simulink model "height_control"  (R2022a)
settings: Solver=VariableStepAuto  StartTime=0.0  StopTime=10.0  RelTol=1e-3
settings Model: Creator=siddh  LastModifiedBy=siddh

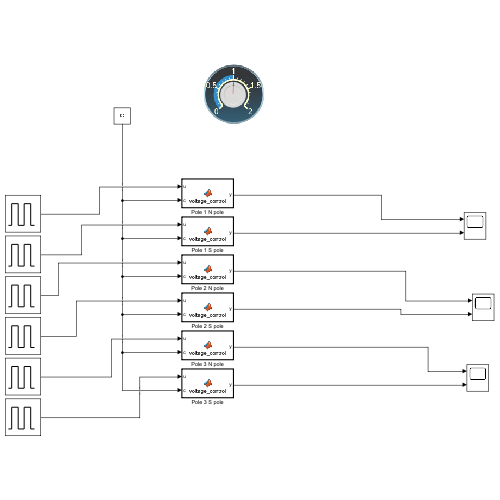
[thumbnail: Simulink's stored preview of the top-level diagram]
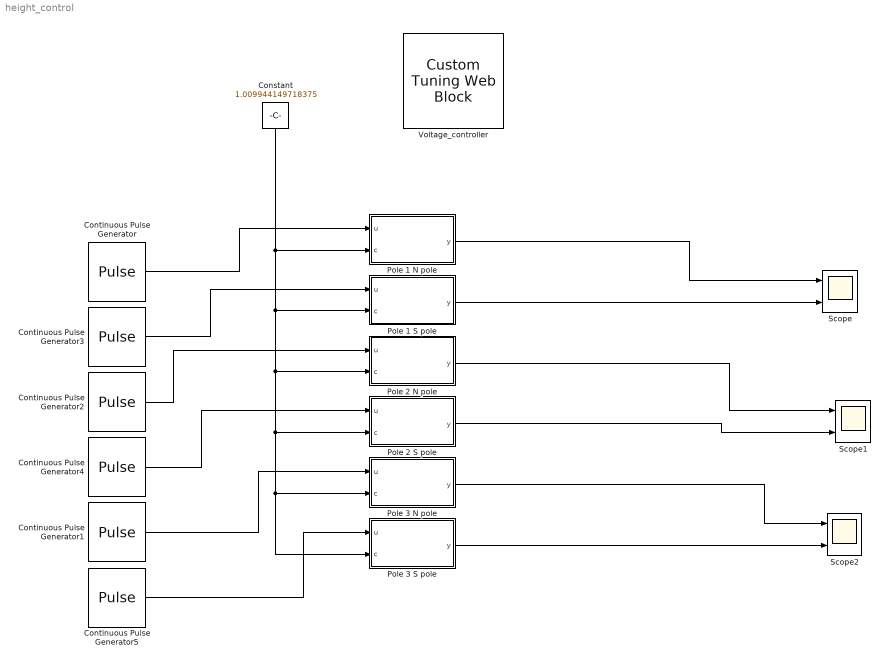
== system height_control ==
  Constant : Constant  Value=1.009944149718375
  Continuous Pulse Generator : DiscretePulseGenerator  PulseType=Time based  Period=3  PulseWidth=100/3
  Continuous Pulse Generator1 : DiscretePulseGenerator  PulseType=Time based  Period=3  PulseWidth=100/3  PhaseDelay=2
  Continuous Pulse Generator2 : DiscretePulseGenerator  PulseType=Time based  Period=3  PulseWidth=100/3  PhaseDelay=1
  Continuous Pulse Generator3 : DiscretePulseGenerator  PulseType=Time based  Amplitude=-1  Period=3  PulseWidth=100/3
  Continuous Pulse Generator4 : DiscretePulseGenerator  PulseType=Time based  Amplitude=-1  Period=3  PulseWidth=100/3  PhaseDelay=1
  Continuous Pulse Generator5 : DiscretePulseGenerator  PulseType=Time based  Amplitude=-1  Period=3  PulseWidth=100/3  PhaseDelay=2
  Pole 1 N pole : MATLAB Function  TreatAsAtomicUnit=on
  Pole 1 S pole : MATLAB Function  TreatAsAtomicUnit=on
  Pole 2 N pole : MATLAB Function  TreatAsAtomicUnit=on
  Pole 2 S pole : MATLAB Function  TreatAsAtomicUnit=on
  Pole 3 N pole : MATLAB Function  TreatAsAtomicUnit=on
  Pole 3 S pole : MATLAB Function  TreatAsAtomicUnit=on
  Scope : Scope  NumInputPorts=2
  Scope1 : Scope  NumInputPorts=2
  Scope2 : Scope  NumInputPorts=2
  Voltage_controller : CustomTuningWebBlock  LabelPosition=Hide  ShowInitialText=on  Configuration="{\"components\":[{\"name\":\"CircularScaleComponent\",\"settings\":{\"bounds\":{\"max\":2,\"min\":0,\"tickInterval\":\"auto\"},\"direction\":\"cw\",\"flipLimits\":0,\"innerRadius\":0.6636618227670849,\"internalTickHeightScaleFactor\":1,\"labelColor\":[255,255,200],\"labelFont\":{\"font\":\"Arial\",\"fontSize\":12},\"labelTransparency\":1,\"minorTickHeightScaleFactor\":0.2,\"needleImage\":{\"size\":[150,150],\"src\":\"data:image\\/svg+xml;base64,PD94bWwgdmVyc2lvbj0iMS4wIiBlbmNvZGluZz0idXRmLTgiPz4NCjwhLS0gR2VuZXJhdG9yOiBBZG9iZSBJbGx1c3RyYXRvciAyNS4yLjMsIFNWRyBFeHBvcnQgUGx1Zy1JbiAuIFNWRyBWZXJzaW9uOiA2LjAwIEJ1aWxkIDApICAtLT4NCjxzdmcgdmVyc2lvbj0iMS4xIiBpZD0iTGF5ZXJfMSIgeG1sbnM9Imh0dHA6Ly93d3cudzMub3JnLzIwMDAvc3ZnIiB4bWxuczp4bGluaz0iaHR0cDovL3d3dy53My5vcmcvMTk5OS94bGluayIgeD0iMHB4IiB5PSIwcHgiDQoJIHZpZXdCb3g9IjAgMCAxNTIgMTUyIiBzdHlsZT0iZW5hYmxl ...(+37472 chars)\"},\"needleOffset\":[0,0],\"needleOrientation\":-45,\"needleRotation\":90,\"needleSize\":{\"height\":0.44,\"width\":0.44},\"outerRadius\":0.5053386200069245,\"position\":[0.004939516129032258,0,1,1],\"referencePoint\":\"auto\",\"scaleAngle\":270,\"scaleAngleOffset\":135,\"scaleColors\":[],\"scaleColorsSize\":0.2,\"scaleDirection\":\"CW\",\"scalePosition\":[0,0,1,1],\"showLabels\":1,\"showMinorTicks\":1,\"showSpanLine\":true,\"showTicks\":1,\"tickColor\":[252,252,197],\"tickTransparency\":1,\"valueBarColor\":[0,114,189],\"valueBarPosition\":[0,0,1,1],\"valueBarSize\":0.2,\"valueBarTransparency\":1}},{\"name\":\"BackgroundImageComponent\",\"settings\":{\"image\":{\"size\":[385,373],\"src\":\"data:image\\/svg+xml;base64,PD94bWwgdmVyc2lvbj0iMS4wIiBlbmNvZGluZz0idXRmLTgiPz4NCjwhLS0gR2VuZXJhdG9yOiBBZG9iZSBJbGx1c3RyYXRvciAyNS4wLjAsIFNWRyBFeHBvcnQgUGx1Zy1JbiAuIFNWRyBWZXJzaW9uOiA2LjAwIEJ1aWxkIDApICAtLT4NCjxzdmcgdmVyc2lvbj0iMS4xIg0KCSBpZD0iTGF5ZXJfMl8xXyIgeG1sbnM6Y2M9Imh0dHA6Ly9jcmVhdGl2ZWNvbW1vbnMub3JnL25zIyIgeG1sbnM6ZGM9Imh0dHA6Ly9wdXJsLm9yZy9kYy9lbGVtZW50cy8xLjEvIiB4bWxuczppbmtzY2FwZT0iaHR0cDovL3d3dy5pbmtzY2FwZS5vcmcv ...(+4184 chars)\",\"srcOrientation\":\"horizontal\"},\"position\":[0,0,1,1],\"scaleMode\":\"0\"}},{\"name\":\"ForegroundImageComponent\",\"settings\":{\"image\":{\"size\":[0,0],\"src\":\"default\",\"srcOrientation\":[]},\"isForeground\":1,\"position\":[0,0,1,1],\"scaleMode\":\"0\"}}],\"settings\":{\"BindingType\":\"param\",\"aspectRatio\":1,\"backgroundColor\":[0,0,0,\"1\"],\"backgroundOffset\":0,\"backgroundOpacity\":1,\"direction\":\"cw\",\"fixedAspectRatio\":\"on\",\"flipLimits\":0,\"foregroundColor\":[252,252,196],\"orientation\":\"horizontal\",\"showBackgroundColor\":false,\"value\":0},\"type\":\"CircularGauge\"}"
  wires:
  Continuous Pulse Generator/1 -> Pole 1 N pole/1(u)
  Pole 1 N pole/1(y) -> Scope/1
  Constant/1 -> Pole 3 S pole/2(c), Pole 3 N pole/2(c), Pole 2 S pole/2(c), Pole 2 N pole/2(c), Pole 1 S pole/2(c), Pole 1 N pole/2(c)
  Continuous Pulse Generator3/1 -> Pole 1 S pole/1(u)
  Pole 1 S pole/1(y) -> Scope/2
  Continuous Pulse Generator2/1 -> Pole 2 N pole/1(u)
  Pole 2 N pole/1(y) -> Scope1/1
  Continuous Pulse Generator4/1 -> Pole 2 S pole/1(u)
  Pole 2 S pole/1(y) -> Scope1/2
  Continuous Pulse Generator1/1 -> Pole 3 N pole/1(u)
  Pole 3 N pole/1(y) -> Scope2/1
  Continuous Pulse Generator5/1 -> Pole 3 S pole/1(u)
  Pole 3 S pole/1(y) -> Scope2/2

== matlab function height_control/Pole 1 N pole ==
  data: u input; y output; c input
function y = voltage_control(u,c)

y = u*c;

end

== matlab function height_control/Pole 2 N pole ==
  data: u input; y output; c input
function y = voltage_control(u,c)

y = u*c;

end

== matlab function height_control/Pole 3 N pole ==
  data: u input; y output; c input
function y = voltage_control(u,c)

y = u*c;

end

== matlab function height_control/Pole 3 S pole ==
  data: u input; y output; c input
function y = voltage_control(u,c)

y = u*c;

end

== matlab function height_control/Pole 2 S pole ==
  data: u input; y output; c input
function y = voltage_control(u,c)

y = u*c;

end

== matlab function height_control/Pole 1 S pole ==
  data: u input; y output; c input
function y = voltage_control(u,c)

y = u*c;

end
